simulink model "sampleModel272"  (R2021b)
settings: Solver=VariableStepAuto  StartTime=0.0  StopTime=10.0  RelTol=1e-3
undefined symbols (not defined in the file or in its folder): DiscIntNeverNeededParam
libraries: simulink x21, slpidlib x4
settings Model: Creator=user  LastModifiedBy=user

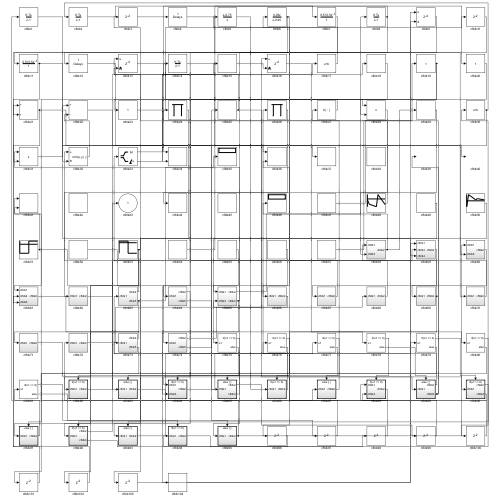
[thumbnail: Simulink's stored preview of the top-level diagram]
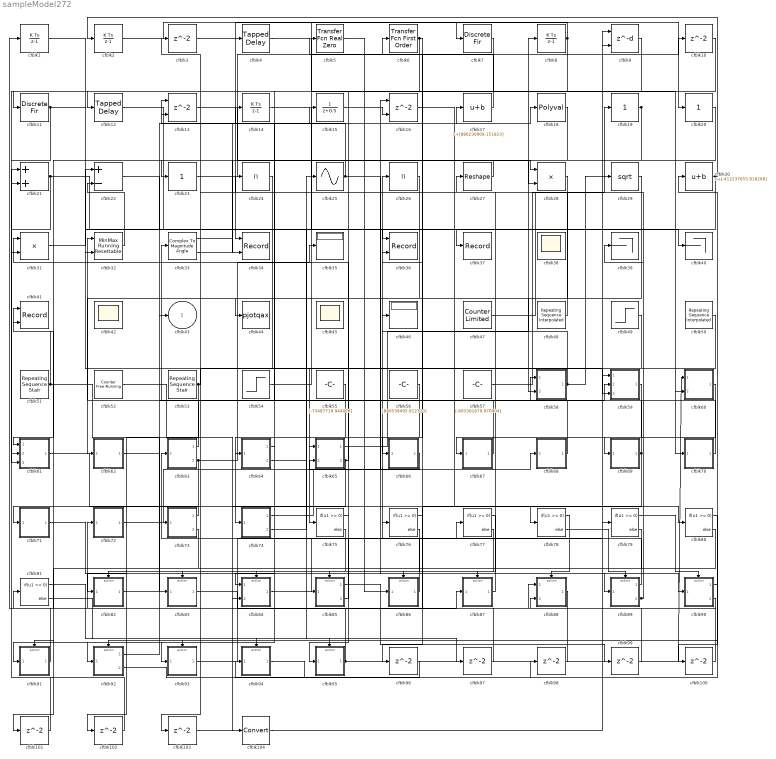
== system sampleModel272 ==
  cfblk{1..2,8,14} (4 alike) : DiscreteIntegrator  ICPrevOutput=DiscIntNeverNeededParam  ICPrevScaledInput=DiscIntNeverNeededParam
  cfblk{3,10,96..103} (10 alike) : Delay  SampleTime=1
  cfblk104 : DataTypeConversion
  cfblk11 : DiscreteFir  SampleTime=1
  cfblk12 : simulink/Discrete/Tapped Delay  vinit=0.0  samptime=-1  NumDelays=1  DelayOrder=Oldest  includeCurrent=off
  cfblk13 : Delay  ShowEnablePort=on  SampleTime=1
      settings: InputPortMap=u0,e6
  cfblk15 : DiscreteTransferFcn  SampleTime=1
  cfblk16 : Delay  ShowEnablePort=on  SampleTime=1
      settings: InputPortMap=u0,e6
  cfblk17 : Bias  Bias=[886230909.151823]
  cfblk18 : Polyval  Coefs=[ +2.081618890e-019, -1.441693666e-014, +4.719686976e-010, -8.536869453e-006, +1.621573104e-001, -8.087801117e+001 ]
  cfblk19 : simulink/Math Operations/Slider Gain  gain=1  low=0  high=2
  cfblk20 : simulink/Math Operations/Slider Gain  gain=1  low=0  high=2
  cfblk21 : Sum
  cfblk22 : Sum  Inputs=+-
  cfblk23 : simulink/Math Operations/Slider Gain  gain=1  low=0  high=2
  cfblk24 : Product  Inputs=*
  cfblk25 : Sin  TimeSource=Use external signal  SampleTime=0
  cfblk26 : Product  Inputs=*
  cfblk27 : Reshape
  cfblk28 : Product  Inputs=**
  cfblk29 : Sqrt  SaturateOnIntegerOverflow=on
  cfblk30 : Bias  Bias=[-412237655.918268]
  cfblk31 : Product  Inputs=**
  cfblk32 : simulink/Math Operations/MinMax Running Resettable  Function=min  vinit=0.0
  cfblk33 : ComplexToMagnitudeAngle
  cfblk34 : Record  FileSettingsInternal="{\"entries\":[{\"content\":{\"excelSettings\":{\"content\":{},\"type\":\"Streamout.ExcelSettings\"}},\"type\":\"Streamout.FileSettingStorage\",\"uuid\":\"0c4fe5c2-4e06-4f9d-937e-dab7eabbd541\"}],\"packageUris\":[\"http://schema.mathworks.com/mf0/streamout_blocks/R2020a\"],\"version\":\"1.0\"}"  Layout=[1 1]  SignalsInternal="{\"entries\":[{\"content\":{\"signals\":[{\"content\":{\"blockPath\":[\"sampleModel272/cfblk34\"],\"channel\":[],\"dimensions\":[1],\"domain\":\"sampleModel272/cfblk34\",\"lineColor\":\"#a2142f\",\"plots\":[1],\"port\":1,\"sid\":[\"\"],\"signalID\":11313,\"signalName\":\"cfblk3\"},\"type\":\"RecordBlkView.Signal\",\"uuid\":\"582825d7-b222-4042-9fc5-050a24171bf2\"},{\"content\":{\"blockPath\":[\"sampleModel272/cfblk34\"],\"channel\":[],\"dimensions\":[1],\"domain\":\"sampleModel272/cfblk34\",\"lineColor\":\"#139fff\",\"plots\":[1],\"port\":2,\"sid\":[\"\"],\"signalID\":11317,\"signalName\":\"cfblk20\"},\"type\":\"RecordBlkView.Signal\",\"uuid\":\"ae994c17-4a30-4e92-9bdf-34956fc0e6cf\"}]},\"type\":\"RecordBlkView.InputSignals\",\"uuid\":\"c3c8f49c-71c0-48e6-ae44-0874ec5f92c6\"}],\"packageUris\":[\"http://schema.mathworks.com/mf0/streamout_blocks/R2020a\"],\"version\":\"1.0\"}"  VisualizationBindings="{\"xyplotplugin\":{\"info\":[{\"series\":[{\"bindingParametersList\":[{\"parameter\":\"X-Axis\",\"signalID\":11313,\"signalName\":\"cfblk3\"},{\"parameter\":\"Y-Axis\",\"signalID\":11317,\"signalName\":\"cfblk20\"}],\"seriesID\":49566}],\"subplotID\":1}]}}"  CompatibilityTag=XY
  cfblk35 : Display
  cfblk36 : Record  FileSettingsInternal="{\"entries\":[{\"content\":{\"excelSettings\":{\"content\":{},\"type\":\"Streamout.ExcelSettings\"}},\"type\":\"Streamout.FileSettingStorage\",\"uuid\":\"e99952ce-eccc-4709-8e11-39aef12f571e\"}],\"packageUris\":[\"http://schema.mathworks.com/mf0/streamout_blocks/R2020a\"],\"version\":\"1.0\"}"  Layout=[1 1]  SignalsInternal="{\"entries\":[{\"content\":{\"signals\":[{\"content\":{\"blockPath\":[\"sampleModel272/cfblk36\"],\"channel\":[],\"dimensions\":[1],\"domain\":\"sampleModel272/cfblk36\",\"lineColor\":\"#a2142f\",\"plots\":[1],\"port\":1,\"sid\":[\"\"],\"signalID\":11293,\"signalName\":\"cfblk22\"},\"type\":\"RecordBlkView.Signal\",\"uuid\":\"389a9882-db56-409b-bae2-0792bad7a1af\"},{\"content\":{\"blockPath\":[\"sampleModel272/cfblk36\"],\"channel\":[],\"dimensions\":[1],\"domain\":\"sampleModel272/cfblk36\",\"lineColor\":\"#139fff\",\"plots\":[1],\"port\":2,\"sid\":[\"\"],\"signalID\":11297,\"signalName\":\"cfblk69\"},\"type\":\"RecordBlkView.Signal\",\"uuid\":\"c88e69b6-a2aa-400e-b828-1db8bb81a6ca\"}]},\"type\":\"RecordBlkView.InputSignals\",\"uuid\":\"921f4008-ae4e-4df1-9e60-ab937aeb3a74\"}],\"packageUris\":[\"http://schema.mathworks.com/mf0/streamout_blocks/R2020a\"],\"version\":\"1.0\"}"  VisualizationBindings="{\"xyplotplugin\":{\"info\":[{\"series\":[{\"bindingParametersList\":[{\"parameter\":\"X-Axis\",\"signalID\":11293,\"signalName\":\"cfblk22\"},{\"parameter\":\"Y-Axis\",\"signalID\":11297,\"signalName\":\"cfblk69\"}],\"seriesID\":34702}],\"subplotID\":1}]}}"  CompatibilityTag=XY
  cfblk37 : Record  FileSettingsInternal="{\"entries\":[{\"content\":{\"excelSettings\":{\"content\":{},\"type\":\"Streamout.ExcelSettings\"}},\"type\":\"Streamout.FileSettingStorage\",\"uuid\":\"df2f9316-2949-4e6a-b5f1-9290091e9f5e\"}],\"packageUris\":[\"http://schema.mathworks.com/mf0/streamout_blocks/R2020a\"],\"version\":\"1.0\"}"  SignalsInternal="{\"entries\":[{\"content\":{\"signals\":[{\"content\":{\"blockPath\":[\"sampleModel272/cfblk37\"],\"channel\":[],\"dimensions\":[1],\"domain\":\"sampleModel272/cfblk37\",\"lineColor\":\"#ff13a6\",\"plots\":[1],\"port\":1,\"sid\":[\"\"],\"signalID\":11301,\"signalName\":\"cfblk11\"},\"type\":\"RecordBlkView.Signal\",\"uuid\":\"6510932c-312c-4101-bbf6-69dbfc47c493\"}]},\"type\":\"RecordBlkView.InputSignals\",\"uuid\":\"95ebdce7-5aef-48e1-80c8-d5cd340afcd3\"}],\"packageUris\":[\"http://schema.mathworks.com/mf0/streamout_blocks/R2020a\"],\"version\":\"1.0\"}"  VisualizationBindings="{\"sparklinesplugin\":{\"info\":[{\"bindingParametersList\":[],\"subplotID\":1}]}}"
  cfblk38 : Scope
      settings: Floating=on
  cfblk39 : Terminator
  cfblk4 : simulink/Discrete/Tapped Delay  vinit=0.0  samptime=-1  NumDelays=1  DelayOrder=Oldest  includeCurrent=off
  cfblk40 : Terminator
  cfblk41 : Record  FileSettingsInternal="{\"entries\":[{\"content\":{\"excelSettings\":{\"content\":{},\"type\":\"Streamout.ExcelSettings\"}},\"type\":\"Streamout.FileSettingStorage\",\"uuid\":\"d05200f3-4bf8-43f1-8025-f599cfe7f558\"}],\"packageUris\":[\"http://schema.mathworks.com/mf0/streamout_blocks/R2020a\"],\"version\":\"1.0\"}"  Layout=[1 1]  SignalsInternal="{\"entries\":[{\"content\":{\"signals\":[{\"content\":{\"blockPath\":[\"sampleModel272/cfblk41\"],\"channel\":[],\"dimensions\":[1],\"domain\":\"sampleModel272/cfblk41\",\"lineColor\":\"#a2142f\",\"plots\":[1],\"port\":1,\"sid\":[\"\"],\"signalID\":11305,\"signalName\":\"cfblk51\"},\"type\":\"RecordBlkView.Signal\",\"uuid\":\"ae742433-c7a0-4431-bb8d-10d0f49611ae\"},{\"content\":{\"blockPath\":[\"sampleModel272/cfblk41\"],\"channel\":[],\"dimensions\":[1],\"domain\":\"sampleModel272/cfblk41\",\"lineColor\":\"#139fff\",\"plots\":[1],\"port\":2,\"sid\":[\"\"],\"signalID\":11309,\"signalName\":\"cfblk95\"},\"type\":\"RecordBlkView.Signal\",\"uuid\":\"d171c5f0-47fc-411c-9592-37ded8902e06\"}]},\"type\":\"RecordBlkView.InputSignals\",\"uuid\":\"820b1682-6594-4112-b81b-05e7c109c2d2\"}],\"packageUris\":[\"http://schema.mathworks.com/mf0/streamout_blocks/R2020a\"],\"version\":\"1.0\"}"  VisualizationBindings="{\"xyplotplugin\":{\"info\":[{\"series\":[{\"bindingParametersList\":[{\"parameter\":\"X-Axis\",\"signalID\":11305,\"signalName\":\"cfblk51\"},{\"parameter\":\"Y-Axis\",\"signalID\":11309,\"signalName\":\"cfblk95\"}],\"seriesID\":56533}],\"subplotID\":1}]}}"  CompatibilityTag=XY
  cfblk42 : Scope
      settings: Floating=on
  cfblk44 : ToWorkspace  VariableName=pjotqax  SaveFormat=Timeseries  SampleTime=-1
  cfblk45 : Scope
      settings: Floating=on
  cfblk46 : Display
  cfblk47 : simulink/Sources/Counter Limited  uplimit=[224.000000]  tsamp=-1
  cfblk48 : simulink/Sources/Repeating Sequence Interpolated  OutValues=[-74356320.899769, -631478197.844560, -900007438.554548, 533032462.067626, -665108209.528397]  TimeValues=[0 0.1 0.5 0.6 1].'  LookUpMeth=Interpolation-Use End Values  tsamp=0.01  OutMin=[]  OutMax=[]  OutDataTypeStr=double  OutputDataTypeScalingMode=double  OutDataType=fixdt(0,8)  OutScaling=2^-10
  cfblk49 : Step  Time=[1.000000]  Before=[-482900987.918856]  After=[568569485.083474]  SampleTime=0
  cfblk5 : simulink/Discrete/Transfer Fcn Real Zero  ZeroZ=0.75  ICPrevInput=0.0  DoSatur=off
      settings: SourceProductBaseCode=SL
  cfblk50 : simulink/Sources/Repeating Sequence Interpolated  OutValues=[-867748794.484662, 985235142.007193, 155666945.266124, 343884439.699508, 169908962.464690]  TimeValues=[0 0.1 0.5 0.6 1].'  LookUpMeth=Use Input Above  tsamp=0.01  OutMin=[]  OutMax=[]  OutDataTypeStr=double  OutputDataTypeScalingMode=double  OutDataType=fixdt(0,8)  OutScaling=2^-10
  cfblk51 : simulink/Sources/Repeating Sequence Stair  OutValues=[-353925477.816012, 121422898.809728]  tsamp=-1  OutMin=[]  OutMax=[]  OutDataTypeStr=double  OutputDataTypeScalingMode=double  OutDataType=fixdt(0,8)  ConRadixGroup=Best Precision: Vector-wise  OutScaling=2^-12
  cfblk52 : simulink/Sources/Counter Free-Running  NumBits=[3.000000]  tsamp=-1
  cfblk53 : simulink/Sources/Repeating Sequence Stair  OutValues=[59744384.389068, -416313144.633542]  tsamp=-1  OutMin=[]  OutMax=[]  OutDataTypeStr=double  OutputDataTypeScalingMode=double  OutDataType=fixdt(0,8)  ConRadixGroup=Best Precision: Vector-wise  OutScaling=2^-12
  cfblk54 : Step  Time=[29.000000]  Before=[118413935.850331]  After=[-954907969.743222]  SampleTime=0
  cfblk55 : Constant  Value=[-73487719.944077]  SampleTime=1
  cfblk56 : Constant  Value=[840539495.912320]  SampleTime=1
  cfblk57 : Constant  Value=[-693301679.970904]  SampleTime=1
  cfblk58 : Subsystem
  cfblk59 : Subsystem
  cfblk6 : simulink/Discrete/Transfer Fcn First Order  PoleZ=0.95  ICPrevOutput=0.0  DoSatur=off
  cfblk60 : Subsystem
  cfblk61 : Subsystem
  cfblk62 : Subsystem
  cfblk63 : Subsystem
  cfblk64 : Subsystem
  cfblk65 : Subsystem
  cfblk66 : Subsystem
  cfblk67 : Subsystem
  cfblk68 : Subsystem
  cfblk69 : Subsystem
  cfblk7 : DiscreteFir  SampleTime=1
  cfblk70 : Subsystem
  cfblk71 : Subsystem
  cfblk72 : Subsystem
  cfblk73 : Subsystem
  cfblk74 : Subsystem
  cfblk{75..81} (7 alike) : If  IfExpression=u1 >= 0  SampleTime=1
  cfblk82 : Subsystem  TreatAsAtomicUnit=on
  cfblk83 : Subsystem  TreatAsAtomicUnit=on
  cfblk84 : Subsystem  TreatAsAtomicUnit=on
  cfblk85 : Subsystem  TreatAsAtomicUnit=on
  cfblk86 : Subsystem  TreatAsAtomicUnit=on
  cfblk87 : Subsystem  TreatAsAtomicUnit=on
  cfblk88 : Subsystem  TreatAsAtomicUnit=on
  cfblk89 : Subsystem  TreatAsAtomicUnit=on
  cfblk9 : Delay  DelayLengthSource=Input port  SampleTime=1
      settings: InputPortMap=u0,p1
  cfblk90 : Subsystem  TreatAsAtomicUnit=on
  cfblk91 : Subsystem  TreatAsAtomicUnit=on
  cfblk92 : Subsystem  TreatAsAtomicUnit=on
  cfblk93 : Subsystem  TreatAsAtomicUnit=on
  cfblk94 : Subsystem  TreatAsAtomicUnit=on
  cfblk95 : Subsystem  TreatAsAtomicUnit=on
  cfblk43 : Outport
  wires:
  cfblk5/1 -> cfblk86/1(cfblk1)
  cfblk54/1 -> cfblk20/1
  cfblk73/1(cfblk2) -> cfblk71/1(cfblk1)
  cfblk88/1(cfblk2) -> cfblk72/1(cfblk1)
  cfblk91/1(cfblk2) -> cfblk1/1
  cfblk95/1(cfblk2) -> cfblk60/1(cfblk1), cfblk41/2
  cfblk14/1 -> cfblk40/1
  cfblk67/1(cfblk2) -> cfblk32/1
  cfblk72/1(cfblk2) -> cfblk68/1(cfblk1)
  cfblk53/1 -> cfblk92/1(cfblk1), cfblk82/1(cfblk1), cfblk13/1
  cfblk13/1 -> cfblk28/1
  cfblk61/1(cfblk2) -> cfblk78/1
  cfblk50/1 -> cfblk75/1
  cfblk93/1(cfblk2) -> cfblk77/1
  cfblk57/1 -> cfblk19/1
  cfblk86/1(cfblk2) -> cfblk26/1
  cfblk83/1(cfblk2) -> cfblk87/1(cfblk1)
  cfblk63/1(cfblk2) -> cfblk33/1
  cfblk89/1(cfblk2) -> cfblk63/1(cfblk1)
  cfblk19/1 -> cfblk28/2, cfblk61/1(cfblk1)
  cfblk30/1 -> cfblk2/1, cfblk32/2
  cfblk59/1(cfblk2) -> cfblk67/1(cfblk1)
  cfblk71/1(cfblk2) -> cfblk90/1(cfblk1)
  cfblk25/1 -> cfblk89/1(cfblk1), cfblk13/2
  cfblk60/1(cfblk2) -> cfblk69/1(cfblk1)
  cfblk8/1 -> cfblk95/1(cfblk1), cfblk4/1
  cfblk84/1(cfblk2) -> cfblk59/1(cfblk1)
  cfblk2/1 -> cfblk7/1
  cfblk63/2(cfblk5) -> cfblk35/1, cfblk102/1
  cfblk12/1 -> cfblk85/1(cfblk1)
  cfblk62/1(cfblk2) -> cfblk59/2(cfblk3)
  cfblk74/1(cfblk2) -> cfblk16/1
  cfblk55/1 -> cfblk65/1(cfblk1)
  cfblk29/1 -> cfblk62/1(cfblk1)
  cfblk68/1(cfblk2) -> cfblk58/1(cfblk1)
  cfblk58/1(cfblk2) -> cfblk46/1, cfblk29/1
  cfblk27/1 -> cfblk23/1
  cfblk23/1 -> cfblk10/1
  cfblk3/1 -> cfblk34/1
  cfblk10/1 -> cfblk12/1
  cfblk21/1 -> cfblk60/2(cfblk5), cfblk61/3(cfblk5)
  cfblk70/1(cfblk2) -> cfblk14/1
  cfblk87/1(cfblk2) -> cfblk27/1
  cfblk94/1(cfblk2) -> cfblk30/1
  cfblk7/1 -> cfblk11/1
  cfblk49/1 -> cfblk93/1(cfblk1)
  cfblk33/1 -> cfblk17/1
  cfblk18/1 -> cfblk84/1(cfblk1)
  cfblk47/1 -> cfblk9/2
  cfblk20/1 -> cfblk34/2
  cfblk11/1 -> cfblk37/1, cfblk31/2
  cfblk66/1(cfblk2) -> cfblk65/2(cfblk3)
  cfblk92/1(cfblk2) -> cfblk43/1
  cfblk31/1 -> cfblk22/1
  cfblk51/1 -> cfblk83/1(cfblk1), cfblk41/1
  cfblk33/2 -> cfblk15/1
  cfblk85/2(cfblk4) -> cfblk73/1(cfblk1)
  cfblk48/1 -> cfblk3/1
  cfblk4/1 -> cfblk70/1(cfblk1)
  cfblk64/1(cfblk2) -> cfblk91/1(cfblk1)
  cfblk89/2(cfblk5) -> cfblk39/1, cfblk24/1
  cfblk17/1 -> cfblk5/1
  cfblk32/1 -> cfblk22/2
  cfblk69/1(cfblk2) -> cfblk36/2, cfblk96/1
  cfblk26/1 -> cfblk44/1
  cfblk16/1 -> cfblk80/1
  cfblk28/1 -> cfblk58/2(cfblk3)
  cfblk90/2(cfblk4) -> cfblk81/1
  cfblk22/1 -> cfblk36/1
  cfblk74/2(cfblk5) -> cfblk25/1
  cfblk56/1 -> cfblk74/1(cfblk1)
  cfblk82/1(cfblk2) -> cfblk18/1
  cfblk6/1 -> cfblk66/1(cfblk1), cfblk64/1(cfblk1)
  cfblk1/1 -> cfblk59/3(cfblk4)
  cfblk9/1 -> cfblk21/2
  cfblk15/1 -> cfblk16/2
  cfblk65/1(cfblk2) -> cfblk8/1
  cfblk65/2(cfblk4) -> cfblk84/2(cfblk3), cfblk31/1
  cfblk75/1 -> cfblk82/Action
  cfblk75/2 -> cfblk83/Action
  cfblk76/1 -> cfblk84/Action
  cfblk76/2 -> cfblk85/Action
  cfblk77/1 -> cfblk86/Action
  cfblk77/2 -> cfblk87/Action
  cfblk78/1 -> cfblk88/Action
  cfblk78/2 -> cfblk89/Action
  cfblk79/1 -> cfblk90/Action
  cfblk79/2 -> cfblk91/Action
  cfblk80/1 -> cfblk92/Action
  cfblk80/2 -> cfblk93/Action
  cfblk81/1 -> cfblk94/Action
  cfblk81/2 -> cfblk95/Action
  cfblk96/1 -> cfblk94/1(cfblk1)
  cfblk64/2(cfblk5) -> cfblk97/1
  cfblk97/1 -> cfblk6/1
  cfblk92/2(cfblk4) -> cfblk98/1
  cfblk98/1 -> cfblk88/2(cfblk3)
  cfblk85/1(cfblk2) -> cfblk99/1
  cfblk99/1 -> cfblk76/1
  cfblk90/1(cfblk2) -> cfblk100/1
  cfblk100/1 -> cfblk88/1(cfblk1)
  cfblk73/2(cfblk5) -> cfblk101/1
  cfblk101/1 -> cfblk21/1
  cfblk102/1 -> cfblk61/2(cfblk4)
  cfblk24/1 -> cfblk103/1
  cfblk103/1 -> cfblk9/1
  cfblk52/1 -> cfblk104/1
  cfblk104/1 -> cfblk79/1

== system sampleModel272/cfblk58 ==
  cfblk1 : Inport
  cfblk3 : Inport  Port=2
  cfblk2 : Outport
  wires:
  cfblk3/1 -> cfblk2/1

== system sampleModel272/cfblk59 ==
  cfblk1 : Inport
  cfblk3 : Inport  Port=2
  cfblk4 : Inport  Port=3
  cfblk2 : Outport
  wires:
  cfblk1/1 -> cfblk2/1

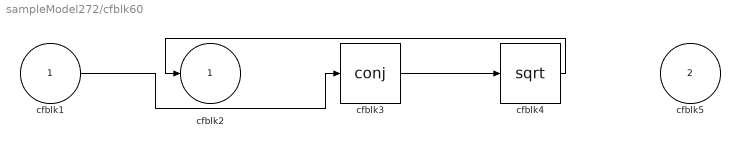
== system sampleModel272/cfblk60 ==
  cfblk1 : Inport
  cfblk5 : Inport  Port=2
  cfblk3 : Math  Operator=conj  SaturateOnIntegerOverflow=on
  cfblk4 : Sqrt  SaturateOnIntegerOverflow=on
  cfblk2 : Outport
  wires:
  cfblk4/1 -> cfblk2/1
  cfblk3/1 -> cfblk4/1
  cfblk1/1 -> cfblk3/1

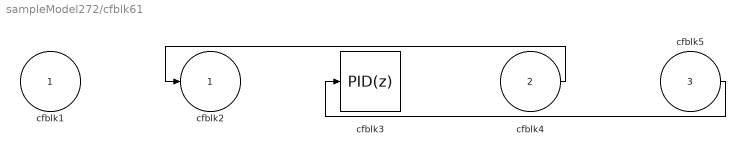
== system sampleModel272/cfblk61 ==
  cfblk1 : Inport
  cfblk4 : Inport  Port=2
  cfblk5 : Inport  Port=3
  cfblk3 : slpidlib/PID Controller  Controller=PID  Form=Parallel  TimeDomain=Discrete-time  UseExternalTs=off  SampleTime=1  IntegratorMethod=Forward Euler  FilterMethod=Forward Euler  ControllerParametersSource=internal  P=1  I=1  D=0  UseFilter=on  N=100  TunerSelectOption=Transfer Function Based (PID Tuner App)  InitialConditionSource=internal  InitialConditionForIntegrator=0  InitialConditionForFilter=0  DifferentiatorICPrevScaledInput=0  ExternalReset=none  TrackingMode=off  Kt=1  LimitOutput=off  SatLimitsSource=internal  UpperSaturationLimit=inf  LowerSaturationLimit=-inf  LinearizeAsGain=off  AntiWindupMode=none  Kb=1  POutMin=[]  POutMax=[]  IOutMin=[]  IOutMax=[]  DOutMin=[]  DOutMax=[]  NOutMin=[]  NOutMax=[]  SumOutMin=[]  SumOutMax=[]  SaturationOutMin=[]  SaturationOutMax=[]  PParamMin=[]  PParamMax=[]  IParamMin=[]  IParamMax=[]  DParamMin=[]  DParamMax=[]  NParamMin=[]  NParamMax=[]  KbParamMin=[]  KbParamMax=[]  KtParamMin=[]  KtParamMax=[]  KbOutMin=[]  KbOutMax=[]  KtOutMin=[]  KtOutMax=[]  IntegratorOutMin=[]  IntegratorOutMax=[]  FilterOutMin=[]  FilterOutMax=[]  SumI1OutMin=[]  SumI1OutMax=[]  SumI2OutMin=[]  SumI2OutMax=[]  SumI3OutMin=[]  SumI3OutMax=[]  SumI4OutMin=[]  SumI4OutMax=[]  SumDOutMin=[]  SumDOutMax=[]  DifferentiatorOutMin=[]  DifferentiatorOutMax=[]  FilterDiffOutCoefMin=[]  FilterDiffOutCoefMax=[]  ReciprocalOutMin=[]  ReciprocalOutMax=[]  SumDenOutMin=[]  SumDenOutMax=[]  SumNumOutMin=[]  SumNumOutMax=[]  DivideOutMin=[]  DivideOutMax=[]  UdiffTsProdOutMin=[]  UdiffTsProdOutMax=[]  NTsProdOutMin=[]  NTsProdOutMax=[]  UintegralTsProdOutMin=[]  UintegralTsProdOutMax=[]  UngainTsProdOutMin=[]  UngainTsProdOutMax=[]  IntegratorContinuousStateAttributes=''  IntegratorStateMustResolveToSignalObject=off  IntegratorRTWStateStorageClass=Auto  FilterContinuousStateAttributes=''  FilterStateMustResolveToSignalObject=off  FilterRTWStateStorageClass=Auto  ParallelPVariant=InternalParameters  IdealPVariant=Disabled  IVariant=InternalParameters  DVariant=InternalParameters  IntegratorVariant=Discrete  SatVariant=Disabled  AWVariant=Passthrough  PCopyVariant=Disabled  TRVariant=Disabled  FdbkBlocksVariant=Forward  IdealPFdbkVariant=Disabled  SatFdbkVariant=Disabled  DerivativeFilterVariant=ForwardEulerFilter  NVariant=InternalParameters  NCopyVariant=Disabled  FilterICVariant=InternalICsFilter  IntegratorICVariant=InternalICs  ExternalResetVariant=Disabled  TRSumVariant=Passthrough  SumFdbkVariant=Disabled  SumVariant=Sum_PID  TsampFilterVariant=InternalTs  TsampNgainVariant=Passthrough  TsampIntegralVariant=Passthrough  ExternalSaturationOutDataTypeStr=Inherit: Same as second input
  cfblk2 : Outport
  wires:
  cfblk4/1 -> cfblk2/1
  cfblk5/1 -> cfblk3/1

== system sampleModel272/cfblk62 ==
  cfblk1 : Inport
  cfblk3 : MinMax  Function=max
  cfblk4 : Constant  Value=[-3671172.779738]  SampleTime=1
  cfblk2 : Outport
  wires:
  cfblk4/1 -> cfblk2/1
  cfblk1/1 -> cfblk3/1

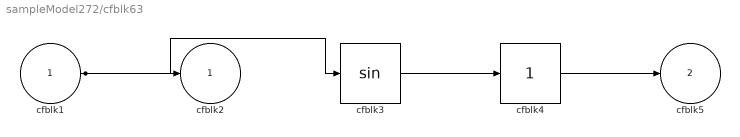
== system sampleModel272/cfblk63 ==
  cfblk1 : Inport
  cfblk3 : Trigonometry
  cfblk4 : simulink/Math Operations/Slider Gain  gain=1  low=0  high=2
  cfblk2 : Outport
  cfblk5 : Outport  Port=2
  wires:
  cfblk4/1 -> cfblk5/1
  cfblk1/1 -> cfblk3/1, cfblk2/1
  cfblk3/1 -> cfblk4/1

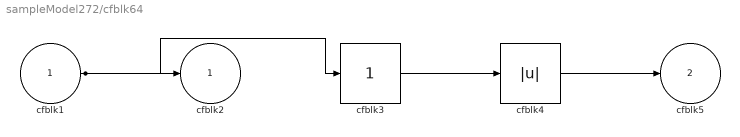
== system sampleModel272/cfblk64 ==
  cfblk1 : Inport
  cfblk3 : simulink/Math Operations/Slider Gain  gain=1  low=0  high=2
  cfblk4 : Abs
  cfblk2 : Outport
  cfblk5 : Outport  Port=2
  wires:
  cfblk4/1 -> cfblk5/1
  cfblk3/1 -> cfblk4/1
  cfblk1/1 -> cfblk2/1, cfblk3/1

== system sampleModel272/cfblk65 ==
  cfblk1 : Inport
  cfblk3 : Inport  Port=2
  cfblk2 : Outport
  cfblk4 : Outport  Port=2
  wires:
  cfblk3/1 -> cfblk2/1
  cfblk1/1 -> cfblk4/1

== system sampleModel272/cfblk66 ==
  cfblk1 : Inport
  cfblk3 : Delay  ShowEnablePort=on  SampleTime=1
      settings: InputPortMap=u0,e6
  cfblk2 : Outport
  wires:
  cfblk1/1 -> cfblk2/1, cfblk3/1, cfblk3/2

== system sampleModel272/cfblk67 ==
  cfblk1 : Inport
  cfblk3 : DiscreteZeroPole  Poles=[0 0.5]  Gain=1
  cfblk4 : simulink/Discrete/Transfer Fcn Lead or Lag  PoleZ=0.95  ZeroZ=0.75  ICPrevOutput=0.0  ICPrevInput=0.0  DoSatur=off
      settings: SourceProductBaseCode=SL
  cfblk2 : Outport
  wires:
  cfblk4/1 -> cfblk2/1
  cfblk3/1 -> cfblk4/1
  cfblk1/1 -> cfblk3/1

== system sampleModel272/cfblk68 ==
  cfblk1 : Inport
  cfblk3 : Polyval  Coefs=[ +2.081618890e-019, -1.441693666e-014, +4.719686976e-010, -8.536869453e-006, +1.621573104e-001, -8.087801117e+001 ]
  cfblk2 : Outport
  wires:
  cfblk1/1 -> cfblk2/1, cfblk3/1

== system sampleModel272/cfblk69 ==
  cfblk1 : Inport
  cfblk3 : Trigonometry
  cfblk2 : Outport
  wires:
  cfblk1/1 -> cfblk3/1
  cfblk3/1 -> cfblk2/1

== system sampleModel272/cfblk70 ==
  cfblk1 : Inport
  cfblk3 : Polyval  Coefs=[ +2.081618890e-019, -1.441693666e-014, +4.719686976e-010, -8.536869453e-006, +1.621573104e-001, -8.087801117e+001 ]
  cfblk2 : Outport
  wires:
  cfblk3/1 -> cfblk2/1
  cfblk1/1 -> cfblk3/1

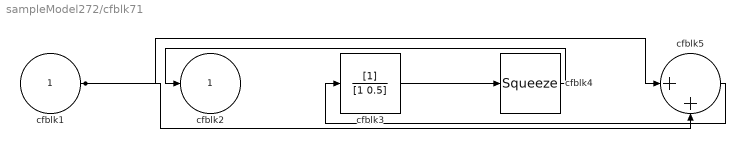
== system sampleModel272/cfblk71 ==
  cfblk1 : Inport
  cfblk3 : DiscreteFilter  SampleTime=1
  cfblk4 : Squeeze
  cfblk5 : Sum  Inputs=|++
  cfblk2 : Outport
  wires:
  cfblk3/1 -> cfblk4/1
  cfblk4/1 -> cfblk2/1
  cfblk5/1 -> cfblk3/1
  cfblk1/1 -> cfblk5/1, cfblk5/2

== system sampleModel272/cfblk72 ==
  cfblk1 : Inport
  cfblk3 : DiscreteIntegrator  ICPrevOutput=DiscIntNeverNeededParam  ICPrevScaledInput=DiscIntNeverNeededParam
  cfblk2 : Outport
  wires:
  cfblk1/1 -> cfblk3/1
  cfblk3/1 -> cfblk2/1

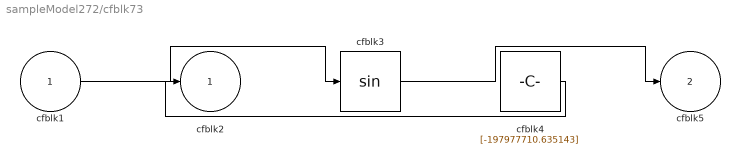
== system sampleModel272/cfblk73 ==
  cfblk1 : Inport
  cfblk3 : Trigonometry
  cfblk4 : Constant  Value=[-197977710.635143]  SampleTime=1
  cfblk2 : Outport
  cfblk5 : Outport  Port=2
  wires:
  cfblk1/1 -> cfblk3/1
  cfblk4/1 -> cfblk2/1
  cfblk3/1 -> cfblk5/1

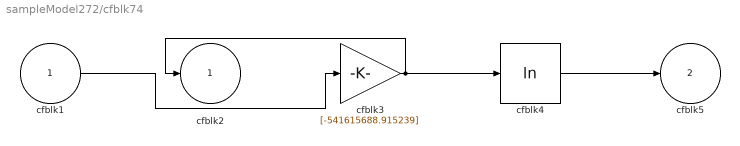
== system sampleModel272/cfblk74 ==
  cfblk1 : Inport
  cfblk3 : Gain  Gain=[-541615688.915239]
  cfblk4 : Math  Operator=log  SaturateOnIntegerOverflow=on
  cfblk2 : Outport
  cfblk5 : Outport  Port=2
  wires:
  cfblk3/1 -> cfblk2/1, cfblk4/1
  cfblk1/1 -> cfblk3/1
  cfblk4/1 -> cfblk5/1

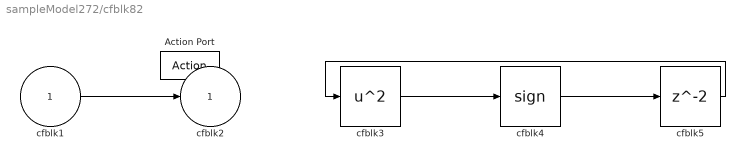
== system sampleModel272/cfblk82 ==
  cfblk1 : Inport
  Action Port : ActionPort  ActionPortLabel=if(u1 >= 0)
  cfblk3 : Math  Operator=square  SaturateOnIntegerOverflow=on
  cfblk4 : Signum
  cfblk5 : Delay
  cfblk2 : Outport
  wires:
  cfblk1/1 -> cfblk2/1
  cfblk3/1 -> cfblk4/1
  cfblk4/1 -> cfblk5/1
  cfblk5/1 -> cfblk3/1

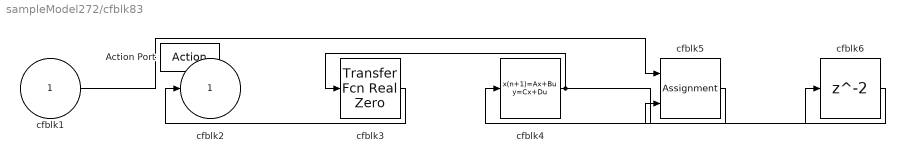
== system sampleModel272/cfblk83 ==
  cfblk1 : Inport
  Action Port : ActionPort  ActionPortLabel=else
  cfblk3 : simulink/Discrete/Transfer Fcn Real Zero  ZeroZ=0.75  ICPrevInput=0.0  DoSatur=off
      settings: SourceProductBaseCode=SL
  cfblk4 : DiscreteStateSpace  SampleTime=-1
  cfblk5 : Assignment  DiagnosticForDimensions=Warning  IndexOptions=Index vector (dialog)  Indices=1  OutputSizes=1
  cfblk6 : Delay
  cfblk2 : Outport
  wires:
  cfblk4/1 -> cfblk3/1, cfblk6/1
  cfblk3/1 -> cfblk2/1
  cfblk5/1 -> cfblk4/1
  cfblk1/1 -> cfblk5/1
  cfblk6/1 -> cfblk5/2

== system sampleModel272/cfblk84 ==
  cfblk1 : Inport
  cfblk3 : Inport  Port=2
  Action Port : ActionPort  ActionPortLabel=if(u1 >= 0)
  cfblk2 : Outport
  wires:
  cfblk1/1 -> cfblk2/1

== system sampleModel272/cfblk85 ==
  cfblk1 : Inport
  Action Port : ActionPort  ActionPortLabel=else
  cfblk3 : DiscreteIntegrator  SampleTime=-1  ICPrevOutput=DiscIntNeverNeededParam  ICPrevScaledInput=DiscIntNeverNeededParam
  cfblk2 : Outport
  cfblk4 : Outport  Port=2
  wires:
  cfblk3/1 -> cfblk2/1, cfblk4/1
  cfblk1/1 -> cfblk3/1

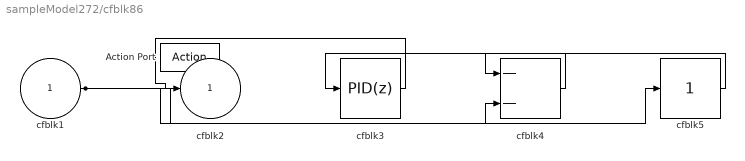
== system sampleModel272/cfblk86 ==
  cfblk1 : Inport
  Action Port : ActionPort  ActionPortLabel=if(u1 >= 0)
  cfblk3 : slpidlib/PID Controller  Controller=PID  Form=Parallel  TimeDomain=Discrete-time  UseExternalTs=off  SampleTime=-1  IntegratorMethod=Forward Euler  FilterMethod=Forward Euler  ControllerParametersSource=internal  P=1  I=1  D=0  UseFilter=on  N=100  TunerSelectOption=Transfer Function Based (PID Tuner App)  InitialConditionSource=internal  InitialConditionForIntegrator=0  InitialConditionForFilter=0  DifferentiatorICPrevScaledInput=0  ExternalReset=none  TrackingMode=off  Kt=1  LimitOutput=off  SatLimitsSource=internal  UpperSaturationLimit=inf  LowerSaturationLimit=-inf  LinearizeAsGain=off  AntiWindupMode=none  Kb=1  POutMin=[]  POutMax=[]  IOutMin=[]  IOutMax=[]  DOutMin=[]  DOutMax=[]  NOutMin=[]  NOutMax=[]  SumOutMin=[]  SumOutMax=[]  SaturationOutMin=[]  SaturationOutMax=[]  PParamMin=[]  PParamMax=[]  IParamMin=[]  IParamMax=[]  DParamMin=[]  DParamMax=[]  NParamMin=[]  NParamMax=[]  KbParamMin=[]  KbParamMax=[]  KtParamMin=[]  KtParamMax=[]  KbOutMin=[]  KbOutMax=[]  KtOutMin=[]  KtOutMax=[]  IntegratorOutMin=[]  IntegratorOutMax=[]  FilterOutMin=[]  FilterOutMax=[]  SumI1OutMin=[]  SumI1OutMax=[]  SumI2OutMin=[]  SumI2OutMax=[]  SumI3OutMin=[]  SumI3OutMax=[]  SumI4OutMin=[]  SumI4OutMax=[]  SumDOutMin=[]  SumDOutMax=[]  DifferentiatorOutMin=[]  DifferentiatorOutMax=[]  FilterDiffOutCoefMin=[]  FilterDiffOutCoefMax=[]  ReciprocalOutMin=[]  ReciprocalOutMax=[]  SumDenOutMin=[]  SumDenOutMax=[]  SumNumOutMin=[]  SumNumOutMax=[]  DivideOutMin=[]  DivideOutMax=[]  UdiffTsProdOutMin=[]  UdiffTsProdOutMax=[]  NTsProdOutMin=[]  NTsProdOutMax=[]  UintegralTsProdOutMin=[]  UintegralTsProdOutMax=[]  UngainTsProdOutMin=[]  UngainTsProdOutMax=[]  IntegratorContinuousStateAttributes=''  IntegratorStateMustResolveToSignalObject=off  IntegratorRTWStateStorageClass=Auto  FilterContinuousStateAttributes=''  FilterStateMustResolveToSignalObject=off  FilterRTWStateStorageClass=Auto  ParallelPVariant=InternalParameters  IdealPVariant=Disabled  IVariant=InternalParameters  DVariant=InternalParameters  IntegratorVariant=Discrete  SatVariant=Disabled  AWVariant=Passthrough  PCopyVariant=Disabled  TRVariant=Disabled  FdbkBlocksVariant=Forward  IdealPFdbkVariant=Disabled  SatFdbkVariant=Disabled  DerivativeFilterVariant=ForwardEulerFilter  NVariant=InternalParameters  NCopyVariant=Disabled  FilterICVariant=InternalICsFilter  IntegratorICVariant=InternalICs  ExternalResetVariant=Disabled  TRSumVariant=Passthrough  SumFdbkVariant=Disabled  SumVariant=Sum_PID  TsampFilterVariant=InternalTs  TsampNgainVariant=Passthrough  TsampIntegralVariant=Passthrough  ExternalSaturationOutDataTypeStr=Inherit: Same as second input
  cfblk4 : Sum  Inputs=--
  cfblk5 : simulink/Math Operations/Slider Gain  gain=1  low=0  high=2
  cfblk2 : Outport
  wires:
  cfblk1/1 -> cfblk5/1, cfblk4/2
  cfblk3/1 -> cfblk2/1
  cfblk5/1 -> cfblk4/1
  cfblk4/1 -> cfblk3/1

== system sampleModel272/cfblk87 ==
  cfblk1 : Inport
  Action Port : ActionPort  ActionPortLabel=else
  cfblk3 : UnitDelay  SampleTime=-1  HasFrameUpgradeWarning=on
  cfblk4 : simulink/Math Operations/MinMax Running Resettable  Function=min  vinit=0.0
  cfblk2 : Outport
  wires:
  cfblk1/1 -> cfblk4/1, cfblk4/2
  cfblk4/1 -> cfblk3/1
  cfblk3/1 -> cfblk2/1

== system sampleModel272/cfblk88 ==
  cfblk1 : Inport
  cfblk3 : Inport  Port=2
  Action Port : ActionPort  ActionPortLabel=if(u1 >= 0)
  cfblk2 : Outport
  wires:
  cfblk1/1 -> cfblk2/1

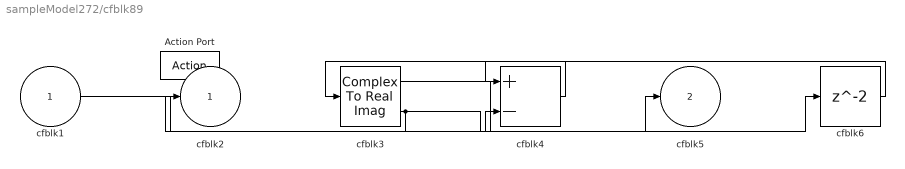
== system sampleModel272/cfblk89 ==
  cfblk1 : Inport
  Action Port : ActionPort  ActionPortLabel=else
  cfblk3 : ComplexToRealImag
  cfblk4 : Sum  Inputs=+-
  cfblk6 : Delay
  cfblk2 : Outport
  cfblk5 : Outport  Port=2
  wires:
  cfblk4/1 -> cfblk3/1
  cfblk3/1 -> cfblk5/1
  cfblk3/2 -> cfblk2/1, cfblk6/1
  cfblk1/1 -> cfblk4/2
  cfblk6/1 -> cfblk4/1

== system sampleModel272/cfblk90 ==
  cfblk1 : Inport
  Action Port : ActionPort  ActionPortLabel=if(u1 >= 0)
  cfblk3 : simulink/Math Operations/MinMax Running Resettable  Function=min  vinit=0.0
  cfblk2 : Outport
  cfblk4 : Outport  Port=2
  wires:
  cfblk1/1 -> cfblk4/1, cfblk3/1, cfblk3/2
  cfblk3/1 -> cfblk2/1

== system sampleModel272/cfblk91 ==
  cfblk1 : Inport
  Action Port : ActionPort  ActionPortLabel=else
  cfblk3 : Gain  Gain=[-75170097.518094]
  cfblk2 : Outport
  wires:
  cfblk1/1 -> cfblk2/1, cfblk3/1

== system sampleModel272/cfblk92 ==
  cfblk1 : Inport
  Action Port : ActionPort  ActionPortLabel=if(u1 >= 0)
  cfblk3 : slpidlib/PID Controller (2DOF)  Controller=PID  Form=Parallel  TimeDomain=Discrete-time  UseExternalTs=off  SampleTime=-1  IntegratorMethod=Forward Euler  FilterMethod=Forward Euler  ControllerParametersSource=internal  P=1  I=1  D=0  UseFilter=on  N=100  b=1  c=1  TunerSelectOption=Transfer Function Based (PID Tuner App)  InitialConditionSource=internal  InitialConditionForIntegrator=0  InitialConditionForFilter=0  DifferentiatorICPrevScaledInput=0  ExternalReset=none  TrackingMode=off  Kt=1  LimitOutput=off  SatLimitsSource=internal  UpperSaturationLimit=inf  LowerSaturationLimit=-inf  LinearizeAsGain=off  AntiWindupMode=none  Kb=1  POutMin=[]  POutMax=[]  IOutMin=[]  IOutMax=[]  DOutMin=[]  DOutMax=[]  NOutMin=[]  NOutMax=[]  bOutMin=[]  bOutMax=[]  cOutMin=[]  cOutMax=[]  SumOutMin=[]  SumOutMax=[]  SaturationOutMin=[]  SaturationOutMax=[]  PParamMin=[]  PParamMax=[]  IParamMin=[]  IParamMax=[]  DParamMin=[]  DParamMax=[]  NParamMin=[]  NParamMax=[]  bParamMin=[]  bParamMax=[]  cParamMin=[]  cParamMax=[]  KbParamMin=[]  KbParamMax=[]  KtParamMin=[]  KtParamMax=[]  KbOutMin=[]  KbOutMax=[]  KtOutMin=[]  KtOutMax=[]  IntegratorOutMin=[]  IntegratorOutMax=[]  FilterOutMin=[]  FilterOutMax=[]  SumI1OutMin=[]  SumI1OutMax=[]  SumI2OutMin=[]  SumI2OutMax=[]  SumI3OutMin=[]  SumI3OutMax=[]  SumI4OutMin=[]  SumI4OutMax=[]  SumDOutMin=[]  SumDOutMax=[]  Sum1OutMin=[]  Sum1OutMax=[]  Sum2OutMin=[]  Sum2OutMax=[]  Sum3OutMin=[]  Sum3OutMax=[]  DifferentiatorOutMin=[]  DifferentiatorOutMax=[]  FilterDiffOutCoefMin=[]  FilterDiffOutCoefMax=[]  ReciprocalOutMin=[]  ReciprocalOutMax=[]  SumDenOutMin=[]  SumDenOutMax=[]  SumNumOutMin=[]  SumNumOutMax=[]  DivideOutMin=[]  DivideOutMax=[]  UdiffTsProdOutMin=[]  UdiffTsProdOutMax=[]  NTsProdOutMin=[]  NTsProdOutMax=[]  UintegralTsProdOutMin=[]  UintegralTsProdOutMax=[]  UngainTsProdOutMin=[]  UngainTsProdOutMax=[]  IntegratorContinuousStateAttributes=''  IntegratorStateMustResolveToSignalObject=off  IntegratorRTWStateStorageClass=Auto  FilterContinuousStateAttributes=''  FilterStateMustResolveToSignalObject=off  FilterRTWStateStorageClass=Auto  ParallelPVariant=InternalParameters  IdealPVariant=Disabled  IVariant=InternalParameters  DVariant=InternalParameters  bVariant=InternalParameters  cVariant=InternalParameters  IntegratorVariant=Discrete  SatVariant=Disabled  AWVariant=Passthrough  PCopyVariant=Disabled  TRVariant=Disabled  FdbkBlocksVariant=Forward  IdealPFdbkVariant=Disabled  SatFdbkVariant=Disabled  DerivativeFilterVariant=ForwardEulerFilter  NVariant=InternalParameters  NCopyVariant=Disabled  FilterICVariant=InternalICsFilter  IntegratorICVariant=InternalICs  ExternalResetVariant=Disabled  TRSumVariant=Passthrough  SumFdbkVariant=Disabled  SumVariant=Sum_PID  TsampFilterVariant=InternalTs  TsampNgainVariant=Passthrough  TsampIntegralVariant=Passthrough  ExternalSaturationOutDataTypeStr=Inherit: Same as second input
      settings: SourceProductBaseCode=SL
  cfblk2 : Outport
  cfblk4 : Outport  Port=2
  wires:
  cfblk1/1 -> cfblk2/1, cfblk3/1, cfblk3/2
  cfblk3/1 -> cfblk4/1

== system sampleModel272/cfblk93 ==
  cfblk1 : Inport
  Action Port : ActionPort  ActionPortLabel=else
  cfblk3 : slpidlib/PID Controller (2DOF)  Controller=PID  Form=Parallel  TimeDomain=Discrete-time  UseExternalTs=off  SampleTime=-1  IntegratorMethod=Forward Euler  FilterMethod=Forward Euler  ControllerParametersSource=internal  P=1  I=1  D=0  UseFilter=on  N=100  b=1  c=1  TunerSelectOption=Transfer Function Based (PID Tuner App)  InitialConditionSource=internal  InitialConditionForIntegrator=0  InitialConditionForFilter=0  DifferentiatorICPrevScaledInput=0  ExternalReset=none  TrackingMode=off  Kt=1  LimitOutput=off  SatLimitsSource=internal  UpperSaturationLimit=inf  LowerSaturationLimit=-inf  LinearizeAsGain=off  AntiWindupMode=none  Kb=1  POutMin=[]  POutMax=[]  IOutMin=[]  IOutMax=[]  DOutMin=[]  DOutMax=[]  NOutMin=[]  NOutMax=[]  bOutMin=[]  bOutMax=[]  cOutMin=[]  cOutMax=[]  SumOutMin=[]  SumOutMax=[]  SaturationOutMin=[]  SaturationOutMax=[]  PParamMin=[]  PParamMax=[]  IParamMin=[]  IParamMax=[]  DParamMin=[]  DParamMax=[]  NParamMin=[]  NParamMax=[]  bParamMin=[]  bParamMax=[]  cParamMin=[]  cParamMax=[]  KbParamMin=[]  KbParamMax=[]  KtParamMin=[]  KtParamMax=[]  KbOutMin=[]  KbOutMax=[]  KtOutMin=[]  KtOutMax=[]  IntegratorOutMin=[]  IntegratorOutMax=[]  FilterOutMin=[]  FilterOutMax=[]  SumI1OutMin=[]  SumI1OutMax=[]  SumI2OutMin=[]  SumI2OutMax=[]  SumI3OutMin=[]  SumI3OutMax=[]  SumI4OutMin=[]  SumI4OutMax=[]  SumDOutMin=[]  SumDOutMax=[]  Sum1OutMin=[]  Sum1OutMax=[]  Sum2OutMin=[]  Sum2OutMax=[]  Sum3OutMin=[]  Sum3OutMax=[]  DifferentiatorOutMin=[]  DifferentiatorOutMax=[]  FilterDiffOutCoefMin=[]  FilterDiffOutCoefMax=[]  ReciprocalOutMin=[]  ReciprocalOutMax=[]  SumDenOutMin=[]  SumDenOutMax=[]  SumNumOutMin=[]  SumNumOutMax=[]  DivideOutMin=[]  DivideOutMax=[]  UdiffTsProdOutMin=[]  UdiffTsProdOutMax=[]  NTsProdOutMin=[]  NTsProdOutMax=[]  UintegralTsProdOutMin=[]  UintegralTsProdOutMax=[]  UngainTsProdOutMin=[]  UngainTsProdOutMax=[]  IntegratorContinuousStateAttributes=''  IntegratorStateMustResolveToSignalObject=off  IntegratorRTWStateStorageClass=Auto  FilterContinuousStateAttributes=''  FilterStateMustResolveToSignalObject=off  FilterRTWStateStorageClass=Auto  ParallelPVariant=InternalParameters  IdealPVariant=Disabled  IVariant=InternalParameters  DVariant=InternalParameters  bVariant=InternalParameters  cVariant=InternalParameters  IntegratorVariant=Discrete  SatVariant=Disabled  AWVariant=Passthrough  PCopyVariant=Disabled  TRVariant=Disabled  FdbkBlocksVariant=Forward  IdealPFdbkVariant=Disabled  SatFdbkVariant=Disabled  DerivativeFilterVariant=ForwardEulerFilter  NVariant=InternalParameters  NCopyVariant=Disabled  FilterICVariant=InternalICsFilter  IntegratorICVariant=InternalICs  ExternalResetVariant=Disabled  TRSumVariant=Passthrough  SumFdbkVariant=Disabled  SumVariant=Sum_PID  TsampFilterVariant=InternalTs  TsampNgainVariant=Passthrough  TsampIntegralVariant=Passthrough  ExternalSaturationOutDataTypeStr=Inherit: Same as second input
      settings: SourceProductBaseCode=SL
  cfblk4 : Constant  Value=[145841654.233063]  SampleTime=1
  cfblk2 : Outport
  wires:
  cfblk3/1 -> cfblk2/1
  cfblk1/1 -> cfblk3/1
  cfblk4/1 -> cfblk3/2

== system sampleModel272/cfblk94 ==
  cfblk1 : Inport
  Action Port : ActionPort  ActionPortLabel=if(u1 >= 0)
  cfblk3 : DiscreteZeroPole  Poles=[0 0.5]  Gain=1  SampleTime=-1
  cfblk2 : Outport
  wires:
  cfblk1/1 -> cfblk3/1
  cfblk3/1 -> cfblk2/1

== system sampleModel272/cfblk95 ==
  cfblk1 : Inport
  Action Port : ActionPort  ActionPortLabel=else
  cfblk3 : Constant  Value=[-47049902.789821]  SampleTime=1
  cfblk2 : Outport
  wires:
  cfblk3/1 -> cfblk2/1
